simulink model "pwm_w_control_modified_version"  (R2019b)
settings: Solver=VariableStepAuto  StartTime=0.0  StopTime=10  RelTol=1e-3
undefined symbols (not defined in the file): sigbuilder_block
libraries: powerlib x10, simulink x5, powerlib_meascontrol x1
settings Model: Creator=82309  LastModifiedBy=82309
settings SolverCC: ZeroCrossAlgorithm=Adaptive
settings DebuggingCC: IgnoredZcDiagnostic=none

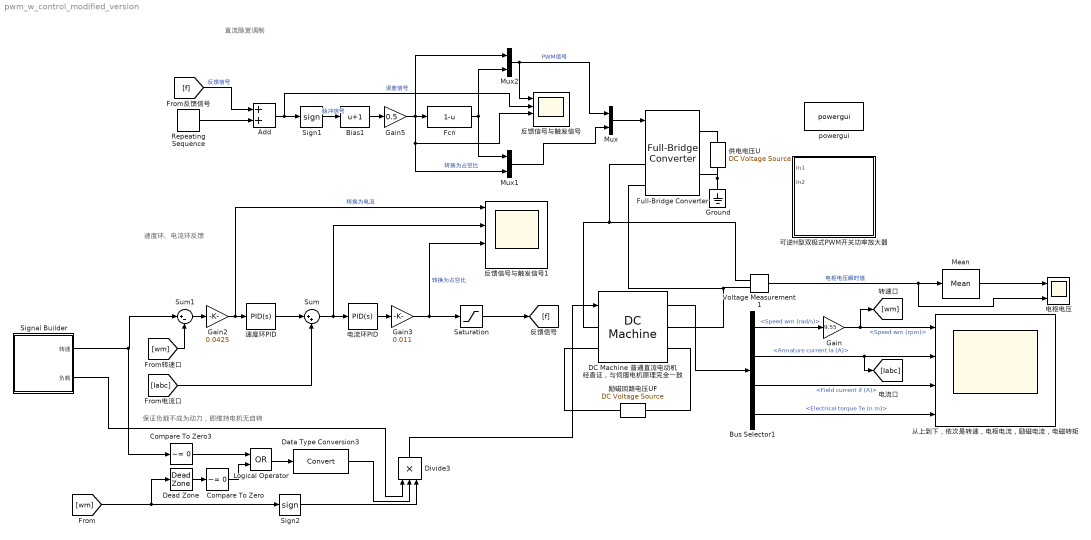
== system pwm_w_control_modified_version ==
  note: 直流脉宽调制
  note: 保证负载不成为动力，即维持电机无自转
  note: 速度环、电流环反馈
  Add : Sum
  Bias1 : Bias  Bias=1
  Bus Selector1 : BusSelector  OutputSignals=Speed wm (rad/s),Armature current ia (A),Field current if (A),Electrical torque Te (n m)
  Compare To Zero : simulink/Logic and Bit Operations/Compare To Zero  relop=~=  OutDataTypeStr=boolean
  Compare To Zero3 : simulink/Logic and Bit Operations/Compare To Zero  relop=~=  OutDataTypeStr=boolean
  DC Machine 普通直流电动机 经查证，与伺服电机原理完全一致 : powerlib/Machines/DC Machine  PresetModel=01: 5HP 240V 1750RPM Field:300V  MechanicalLoad=Torque TL  FieldType=Wound  ShowDetailedParameters=on  MeasurementBus=off  RLa=[2.581 0.028]  RLf=[281.3 156]  Laf=0.9483  MachineConstant=Torque constant (N.m/A)  Ke=1.8  Kt=1.8  J=0.02215  Bm=0.002953  Tf=0.5161  w0=1  Ifinit=1  TsPowergui=0  TsBlock=-1
      settings: SourceProductName=Simscape Electrical
  Data Type Conversion3 : DataTypeConversion
  Dead Zone : DeadZone  SaturateOnIntegerOverflow=on
  Divide3 : Product  Inputs=***
  Fcn : Fcn  Expr=1-u
  Full-Bridge Converter : powerlib/Power Electronics/Full-Bridge Converter  ModelType=Switching devices  Ron=1e-3  Rs=1e6  Cs=inf  Vforward=[0,0]  Ron_Diode=1e-3  Rs_Diode=1e6  Cs_Diode=inf  Vf_Diode=1e-3  Rs_CurrentSource=inf
      settings: SourceProductName=Simscape Electrical  SourceProductBaseCode=PS
  Gain : Gain  Gain=9.55
  Gain2 : Gain  Gain=0.0425
  Gain3 : Gain  Gain=0.011
  Gain5 : Gain  Gain=0.5
  Ground : powerlib/Elements/Ground  LConnTagsString=a
      settings: SourceProductName=Simscape Electrical
  Logical Operator : Logic  Operator=OR  AllPortsSameDT=off  OutDataTypeStr=boolean
  Mean : powerlib_meascontrol/Measurements/Mean  Freq=60  Vinit=0  Ts=0
      settings: SourceProductName=Simscape Electrical
  Mux : Mux  Inputs=2
  Mux1 : Mux  Inputs=2
  Mux2 : Mux  Inputs=2
  Repeating Sequence : simulink/Sources/Repeating Sequence  rep_seq_t=[0 0.001 0.002]  rep_seq_y=[-1 1 -1]
  Saturation : Saturate  UpperLimit=1  LowerLimit=-1
  Sign1 : Signum
  Sign2 : Signum
  Signal Builder : Subsystem  Tag=STV Subsys  LoadFcn=sigbuilder_block('load');  StartFcn=sigbuilder_block('start');  StopFcn=sigbuilder_block('stop');  ClipboardFcn=sigbuilder_block('clipboard');  mask(Sigbuilder block){tuvar=[0:10]}
      mask help: Sigbuilder GUI
      mask init:
      | if ~strcmp(get_param(bdroot(gcbh),'SimulationStatus'),'stopped') tuvar = sigbuilder_block('maskInit'); end
      settings: CopyFcn=sigbuilder_block('copy');  DeleteFcn=sigbuilder_block('delete');  ModelCloseFcn=sigbuilder_block('modelClose');  PreSaveFcn=sigbuilder_block('preSave');  PauseFcn=sigbuilder_block('pause')  ContinueFcn=sigbuilder_block('continue')  NameChangeFcn=sigbuilder_block('namechange');  OpenFcn=sigbuilder_block('open',[416.4 111 550.8 363.6 ]);  CloseFcn=sigbuilder_block('close');
      mask Display: plot(0, 0, 100, 100,[2, 2, 32, 32, 2], [68, 8, 8, 68, 68],[32, 2], [38, 38], [32, 19, 2],[53, 60, 44], [32, 17, 17, 2],[16, 16, 31, 31]);txt = getActiveGroup(gcbh);text(2, 100, txt,'verticalAlignment', 'top');
  Sum : Sum  Inputs=|++
  Sum1 : Sum  Inputs=|+-
  Voltage Measurement1 : powerlib/Measurements/Voltage Measurement  PhasorSimulation=off  OutputType=Complex  PSBequivalent=0
      settings: SourceProductName=Simscape Electrical
  powergui : powerlib/powergui  Priority=1  SimulationMode=Continuous  SampleTime=50e-6  frequency=60  Iterations=50  frequencyindice=0  Pbase=100e6  ErrMax=1e-4  UnitsV=kV  UnitsW=MW  buscounter=0  FunctionMessages=off  echomessages=off  EnableUseOfTLC=off  CurrentSourceSwitches=off  DisableSnubberDevices=off  DisableRonSwitches=off  DisableVfSwitches=off  DisplayEquations=off  AutomaticDiscreteSolvers=off  SolverType=Tustin/Backward Euler (TBE)  Interpol=off  ExternalGateDelay=off  methode=off  Ts=100  x0status=blocks  SPID=on  SwTol=0  HookPort=off  NonlinearTolerance=1e-4  nMaxIteration=100  ContinueOnMaxIteration=off  RestoreLinks=warning  ResistiveCurrentMeasurement=off  Frange=[0:2:500]  Ylog=off  Xlog=on  ShowGrid=off  save=off  variable=ZData  structure=0  ZoomFFT=off  StartTime=0.0  cycles=1  DisplayStyle=1  fundamental=60  FreqAxis=off  MaxFrequency=1000  frequencyindicesteady=1  RmsSteady=1  display=off
      settings: SourceProductName=Simscape Electrical
  从上到下，依次是转速，电枢电流，励磁电流，电磁转矩 : Scope  NumInputPorts=4
  "供电电压U " : powerlib/Electrical Sources/DC Voltage Source  Amplitude=240  Measurements=None
      settings: SourceProductName=Simscape Electrical
  励磁回路电压UF : powerlib/Electrical Sources/DC Voltage Source  Amplitude=300  Measurements=None
      settings: SourceProductName=Simscape Electrical
  反馈信号与触发信号 : Scope  NumInputPorts=4
  反馈信号与触发信号1 : Scope  NumInputPorts=4
  可逆H型双极式PWM开关功率放大器 : Subsystem
  电枢电压 : Scope  NumInputPorts=3
  电流环PID : simulink/Continuous/PID Controller  Controller=PID  Form=Parallel  TimeDomain=Continuous-time  SampleTime=-1  IntegratorMethod=Forward Euler  FilterMethod=Forward Euler  ControllerParametersSource=internal  P=0.5  I=0  D=0  UseFilter=on  N=100  TunerSelectOption=Transfer Function Based (PID Tuner App)  InitialConditionSource=internal  InitialConditionForIntegrator=0  InitialConditionForFilter=0  DifferentiatorICPrevScaledInput=0  ExternalReset=none  TrackingMode=off  Kt=1  LimitOutput=on  UpperSaturationLimit=240  LowerSaturationLimit=-240  LinearizeAsGain=on  AntiWindupMode=none  Kb=1  POutMin=[]  POutMax=[]  IOutMin=[]  IOutMax=[]  DOutMin=[]  DOutMax=[]  NOutMin=[]  NOutMax=[]  SumOutMin=[]  SumOutMax=[]  SaturationOutMin=[]  SaturationOutMax=[]  PParamMin=[]  PParamMax=[]  IParamMin=[]  IParamMax=[]  DParamMin=[]  DParamMax=[]  NParamMin=[]  NParamMax=[]  KbParamMin=[]  KbParamMax=[]  KtParamMin=[]  KtParamMax=[]  KbOutMin=[]  KbOutMax=[]  KtOutMin=[]  KtOutMax=[]  IntegratorOutMin=[]  IntegratorOutMax=[]  FilterOutMin=[]  FilterOutMax=[]  SumI1OutMin=[]  SumI1OutMax=[]  SumI2OutMin=[]  SumI2OutMax=[]  SumI3OutMin=[]  SumI3OutMax=[]  SumI4OutMin=[]  SumI4OutMax=[]  SumDOutMin=[]  SumDOutMax=[]  DifferentiatorOutMin=[]  DifferentiatorOutMax=[]  FilterDiffOutCoefMin=[]  FilterDiffOutCoefMax=[]  ReciprocalOutMin=[]  ReciprocalOutMax=[]  SumDenOutMin=[]  SumDenOutMax=[]  SumNumOutMin=[]  SumNumOutMax=[]  DivideOutMin=[]  DivideOutMax=[]  IntegratorContinuousStateAttributes=''  IntegratorStateMustResolveToSignalObject=off  IntegratorRTWStateStorageClass=Auto  FilterContinuousStateAttributes=''  FilterStateMustResolveToSignalObject=off  FilterRTWStateStorageClass=Auto  ParallelPVariant=InternalParameters  IdealPVariant=Disabled  IVariant=InternalParameters  DVariant=InternalParameters  IntegratorVariant=Continuous  SatVariant=Enabled  AWVariant=Passthrough  PCopyVariant=Disabled  TRVariant=Disabled  FdbkBlocksVariant=Forward  IdealPFdbkVariant=Disabled  SatFdbkVariant=Disabled  DerivativeFilterVariant=ContFilter  NVariant=InternalParameters  NCopyVariant=Disabled  FilterICVariant=InternalICsFilter  IntegratorICVariant=InternalICs  ExternalResetVariant=Disabled  TRSumVariant=Passthrough  SumFdbkVariant=Disabled  SumVariant=Sum_PID
  速度环PID : simulink/Continuous/PID Controller  Controller=PID  Form=Parallel  TimeDomain=Continuous-time  SampleTime=-1  IntegratorMethod=Forward Euler  FilterMethod=Forward Euler  ControllerParametersSource=internal  P=20000  I=10  D=0  UseFilter=on  N=100  TunerSelectOption=Transfer Function Based (PID Tuner App)  InitialConditionSource=internal  InitialConditionForIntegrator=0  InitialConditionForFilter=0  DifferentiatorICPrevScaledInput=0  ExternalReset=none  TrackingMode=off  Kt=1  LimitOutput=on  UpperSaturationLimit=240  LowerSaturationLimit=-240  LinearizeAsGain=on  AntiWindupMode=none  Kb=1  POutMin=[]  POutMax=[]  IOutMin=[]  IOutMax=[]  DOutMin=[]  DOutMax=[]  NOutMin=[]  NOutMax=[]  SumOutMin=[]  SumOutMax=[]  SaturationOutMin=[]  SaturationOutMax=[]  PParamMin=[]  PParamMax=[]  IParamMin=[]  IParamMax=[]  DParamMin=[]  DParamMax=[]  NParamMin=[]  NParamMax=[]  KbParamMin=[]  KbParamMax=[]  KtParamMin=[]  KtParamMax=[]  KbOutMin=[]  KbOutMax=[]  KtOutMin=[]  KtOutMax=[]  IntegratorOutMin=[]  IntegratorOutMax=[]  FilterOutMin=[]  FilterOutMax=[]  SumI1OutMin=[]  SumI1OutMax=[]  SumI2OutMin=[]  SumI2OutMax=[]  SumI3OutMin=[]  SumI3OutMax=[]  SumI4OutMin=[]  SumI4OutMax=[]  SumDOutMin=[]  SumDOutMax=[]  DifferentiatorOutMin=[]  DifferentiatorOutMax=[]  FilterDiffOutCoefMin=[]  FilterDiffOutCoefMax=[]  ReciprocalOutMin=[]  ReciprocalOutMax=[]  SumDenOutMin=[]  SumDenOutMax=[]  SumNumOutMin=[]  SumNumOutMax=[]  DivideOutMin=[]  DivideOutMax=[]  IntegratorContinuousStateAttributes=''  IntegratorStateMustResolveToSignalObject=off  IntegratorRTWStateStorageClass=Auto  FilterContinuousStateAttributes=''  FilterStateMustResolveToSignalObject=off  FilterRTWStateStorageClass=Auto  ParallelPVariant=InternalParameters  IdealPVariant=Disabled  IVariant=InternalParameters  DVariant=InternalParameters  IntegratorVariant=Continuous  SatVariant=Enabled  AWVariant=Passthrough  PCopyVariant=Disabled  TRVariant=Disabled  FdbkBlocksVariant=Forward  IdealPFdbkVariant=Disabled  SatFdbkVariant=Disabled  DerivativeFilterVariant=ContFilter  NVariant=InternalParameters  NCopyVariant=Disabled  FilterICVariant=InternalICsFilter  IntegratorICVariant=InternalICs  ExternalResetVariant=Disabled  TRSumVariant=Passthrough  SumFdbkVariant=Disabled  SumVariant=Sum_PID
  wires:
  Mux2/1 -> Mux/1, 反馈信号与触发信号/1  "PWM信号"
  Mux1/1 -> Mux/2
  Gain/1 -> [wm], 从上到下，依次是转速，电枢电流，励磁电流，电磁转矩/1  "<Speed wm (rpm)>"
  DC Machine 普通直流电动机 经查证，与伺服电机原理完全一致/1 -> Bus Selector1/1
  Bus Selector1/4 -> 从上到下，依次是转速，电枢电流，励磁电流，电磁转矩/4  "<Electrical torque Te (n m)>"
  Bus Selector1/2 -> [Iabc], 从上到下，依次是转速，电枢电流，励磁电流，电磁转矩/2  "<Armature current ia (A)>"
  Bus Selector1/3 -> 从上到下，依次是转速，电枢电流，励磁电流，电磁转矩/3  "<Field current if (A)>"
  Bus Selector1/1 -> Gain/1  "<Speed wm (rad/s)>"
  Voltage Measurement1/1 -> Mean/1, 电枢电压/3  "电枢电压瞬时值"
  Add/1 -> Sign1/1, 反馈信号与触发信号/2  "误差信号"
  Sign1/1 -> Bias1/1  "脉冲信号"
  Divide3/1 -> DC Machine 普通直流电动机 经查证，与伺服电机原理完全一致/1
  Mux/1 -> Full-Bridge Converter/1
  Fcn/1 -> Mux2/2, Mux1/1
  Repeating Sequence/1 -> Add/2
  [wm] -> Sum1/2
  Sum/1 -> 反馈信号与触发信号1/2, 电流环PID/1
  速度环PID/1 -> Sum/1
  Gain3/1 -> 反馈信号与触发信号1/3, Saturation/1  "转换为占空比"
  Signal Builder/1(转速) -> Compare To Zero3/1, Sum1/1
  Sum1/1 -> Gain2/1
  Gain2/1 -> 反馈信号与触发信号1/1, 速度环PID/1  "转换为电流"
  电流环PID/1 -> Gain3/1
  [Iabc] -> Sum/2
  Saturation/1 -> [f]
  Bias1/1 -> Gain5/1
  Gain5/1 -> Fcn/1, Mux2/1, Mux1/2, 反馈信号与触发信号/3  "转换为占空比"
  Mean/1 -> 电枢电压/1
  [f] -> Add/1  "反馈信号"
  [wm] -> Sign2/1, Dead Zone/1
  Dead Zone/1 -> Compare To Zero/1
  Logical Operator/1 -> Data Type Conversion3/1
  Signal Builder/2(负载) -> Divide3/1
  Sign2/1 -> Divide3/3
  Compare To Zero3/1 -> Logical Operator/1
  Compare To Zero/1 -> Logical Operator/2
  Data Type Conversion3/1 -> Divide3/2
  connections:
  Full-Bridge Converter/RConn2 -- "供电电压U "/LConn1 -- Ground/LConn1
  励磁回路电压UF/RConn1 -- DC Machine 普通直流电动机 经查证，与伺服电机原理完全一致/LConn2
  励磁回路电压UF/LConn1 -- DC Machine 普通直流电动机 经查证，与伺服电机原理完全一致/RConn2
  "供电电压U "/RConn1 -- Full-Bridge Converter/RConn1
  Voltage Measurement1/LConn1 -- Full-Bridge Converter/LConn1 -- DC Machine 普通直流电动机 经查证，与伺服电机原理完全一致/LConn1
  Voltage Measurement1/LConn2 -- Full-Bridge Converter/LConn2 -- DC Machine 普通直流电动机 经查证，与伺服电机原理完全一致/RConn1

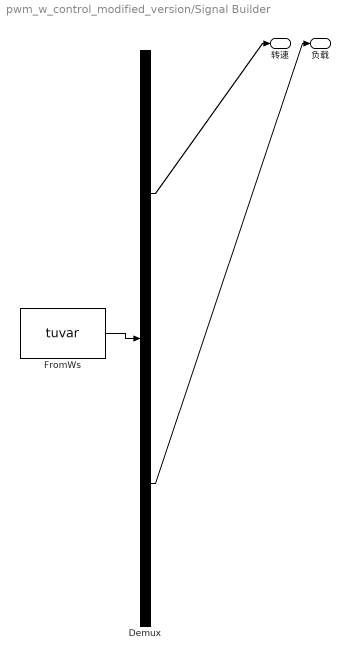
== system pwm_w_control_modified_version/Signal Builder ==
  Demux : Demux  Tag=STV Demux  Outputs=2
  FromWs : FromWorkspace  Tag=STV FromWs  VariableName=tuvar  SampleTime=0
      SigBuilderData=|
      | common.afterFinalStr = 'Extrapolate'
      | common.sampleTime = 0
      | dataSet.timeRange = [0 10]
      | dataSet.name = 'Group 1'
      | sbobj.Groups.Name = 'Group 1'
      | sbobj.Groups.Signals(1).Name = '转速'
      | sbobj.Groups.Signals(1).XData = [0 4.46 4.46 8.48 8.48 10]
      | sbobj.Groups.Signals(1).YData = [1000 1000 -1450 -1450 0 0]
      | sbobj.Groups.Signals(2).Name = '负载'
      | sbobj.Groups.Signals(2).XData = [0 0.5 0.5 1.48 1.48 2.48 2.48 3.49 3.49 5.1 5.1 6.62 6.62 7.72 7.72 10]
      | sbobj.Groups.Signals(2).YData = [0 0 50 50 40 40 29 29 0 0 20.5 20.5 34 34 0 0]
  转速 : Outport  Tag=STV Outport  VectorParamsAs1DForOutWhenUnconnected=off
  负载 : Outport  Tag=STV Outport  Port=2
  wires:
  FromWs/1 -> Demux/1
  Demux/1 -> 转速/1
  Demux/2 -> 负载/1

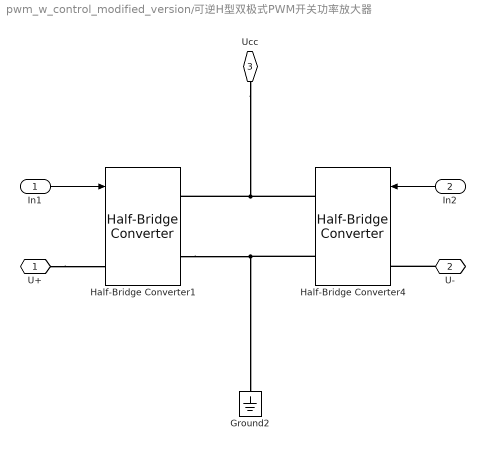
== system pwm_w_control_modified_version/可逆H型双极式PWM开关功率放大器 ==
  In1 : Inport
  In2 : Inport  Port=2
  Ground2 : powerlib/Elements/Ground  LConnTagsString=a
      settings: SourceProductName=Simscape Electrical
  Half-Bridge Converter1 : powerlib/Power Electronics/Half-Bridge Converter  ModelType=Switching devices  Ron=1e-3  Rs=1e6  Cs=inf  Vforward=[0,0]  Ron_Diode=1e-3  Rs_Diode=1e6  Cs_Diode=inf  Vf_Diode=1e-3  Rs_CurrentSource=inf
      settings: SourceProductName=Simscape Electrical  SourceProductBaseCode=PS
  Half-Bridge Converter4 : powerlib/Power Electronics/Half-Bridge Converter  ModelType=Switching devices  Ron=1e-3  Rs=1e6  Cs=inf  Vforward=[0,0]  Ron_Diode=1e-3  Rs_Diode=1e6  Cs_Diode=inf  Vf_Diode=1e-3  Rs_CurrentSource=inf
      settings: SourceProductName=Simscape Electrical  SourceProductBaseCode=PS
  U+ : PMIOPort  Side=Left
  "U- " : PMIOPort  Port=2  Side=Left
  Ucc : PMIOPort  Port=3  Side=Left
  wires:
  In2/1 -> Half-Bridge Converter4/1
  In1/1 -> Half-Bridge Converter1/1
  connections:
  Half-Bridge Converter4/RConn1 -- Ucc/RConn1 -- Half-Bridge Converter1/RConn1
  Half-Bridge Converter1/RConn2 -- Half-Bridge Converter4/RConn2 -- Ground2/LConn1
  U+/RConn1 -- Half-Bridge Converter1/LConn1
  "U- "/RConn1 -- Half-Bridge Converter4/LConn1
